simulink model "y_loop"  (Simulink 8.2)
settings: Solver=ode45  StartTime=0.0  StopTime=50  RelTol=1e-3
undefined symbols (not defined in the file): P
settings Model: Creator=paul  LastModifiedBy=paul
settings DataIOCC: SignalLoggingSaveFormat=Dataset
settings OptimizationCC: ExpressionDepthLimit=128
settings DebuggingCC: FcnCallInpInsideContextMsg=EnableAllAsError  StateNameClashWarn=none
settings GRTTargetCC: CombineOutputUpdateFcns=on  GRTInterface=off

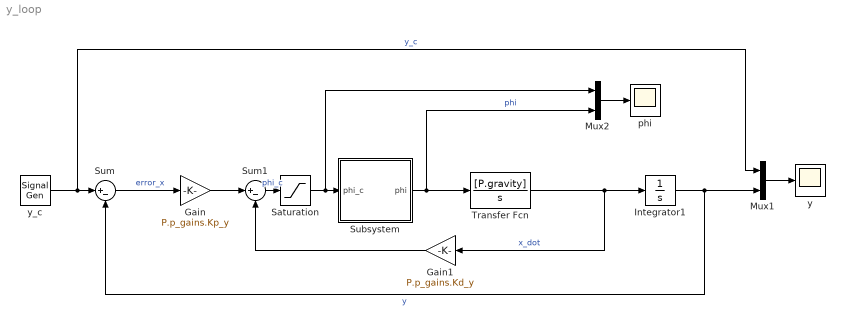
== system y_loop ==
  Gain : Gain  Gain=P.p_gains.Kp_y
  Gain1 : Gain  Gain=P.p_gains.Kd_y
  Integrator1 : Integrator
  Mux1 : Mux  Inputs=2
  Mux2 : Mux  Inputs=2
  Saturation : Saturate  UpperLimit=P.roll_c_max  LowerLimit=-P.roll_c_max
  Subsystem : Subsystem
  Sum : Sum  Inputs=|+-
  Sum1 : Sum  Inputs=|+-
  Transfer Fcn : TransferFcn  Numerator=[P.gravity]  Denominator=[1 0]
  phi : Scope
      settings: YMin=-50  YMax=750
  y : Scope
      settings: TimeRange=50  YMin=-0.4  YMax=0.3  SaveName=ScopeData2
  y_c : SignalGenerator  WaveForm=square  Amplitude=0.25  Frequency=.05
  wires:
  Mux1/1 -> y/1
  y_c/1 -> Mux1/1, Sum/1  "y_c"
  Integrator1/1 -> Mux1/2, Sum/2  "y"
  Gain1/1 -> Sum1/2
  Sum/1 -> Gain/1  "error_x"
  Gain/1 -> Sum1/1
  Mux2/1 -> phi/1
  Transfer Fcn/1 -> Integrator1/1, Gain1/1  "x_dot"
  Sum1/1 -> Saturation/1  "phi_c"
  Subsystem/1(phi) -> Mux2/2, Transfer Fcn/1  "phi"
  Saturation/1 -> Mux2/1, Subsystem/1(phi_c)

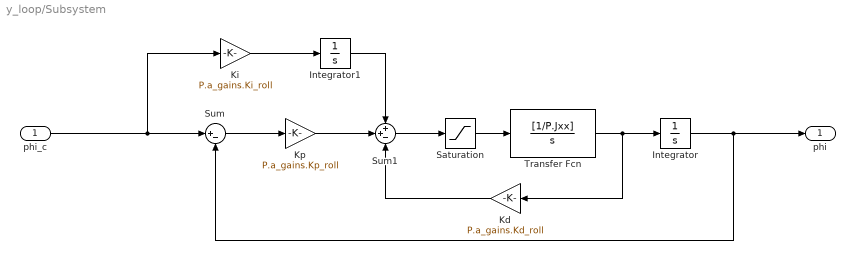
== system y_loop/Subsystem ==
  phi_c : Inport
  Integrator : Integrator
  Integrator1 : Integrator
  Kd : Gain  Gain=P.a_gains.Kd_roll
  Ki : Gain  Gain=P.a_gains.Ki_roll
  Kp : Gain  Gain=P.a_gains.Kp_roll
  Saturation : Saturate
  Sum : Sum  Inputs=|+-
  Sum1 : Sum  Inputs=++-
  Transfer Fcn : TransferFcn  Numerator=[1/P.Jxx]  Denominator=[1 0]
  phi : Outport
  wires:
  Saturation/1 -> Transfer Fcn/1
  Transfer Fcn/1 -> Kd/1, Integrator/1
  Kp/1 -> Sum1/2
  Integrator/1 -> phi/1, Sum/2
  Sum1/1 -> Saturation/1
  Ki/1 -> Integrator1/1
  Sum/1 -> Kp/1
  Integrator1/1 -> Sum1/1
  Kd/1 -> Sum1/3
  phi_c/1 -> Ki/1, Sum/1
